simulink model "QArm_with_Dynamic_Model"  (R2024a)
settings: Solver=ode4  StartTime=0.0  StopTime=inf  FixedStep=1/500  RelTol=1e-3  EnableMultiTasking=on
undefined symbols (not defined in the file): HIL, qc_get_step_size
libraries: quarc_library x13
settings Model: SimulationMode=external  ExtModeTrigDuration=10000  Creator=fvranes  LastModifiedBy=mbohra
settings SolverCC: AlgebraicLoopSolver=TrustRegion  PositivePriorityOrder=on
settings DataIOCC: SaveOutput=off  SignalLogging=off  DSMLogging=off  SaveTime=off  ReturnWorkspaceOutputs=off
settings OptimizationCC: ReuseModelBlockBuffer=off
settings DebuggingCC: UnconnectedInputMsg=warning  UnconnectedOutputMsg=warning  UnconnectedLineMsg=warning  ArithmeticOperatorsInVariantConditions=warning
settings ModelReferenceCC: EnableRefExpFcnMdlSchedulingChecks=on
settings SFSimCC: SimUseLocalCustomCode=off  CustomCodeUndefinedFunction=UseInterfaceOnly
settings RTWCC: Description=QUARC Win64 Target Using Toolchain  SystemTargetFile=quarc_win64.tlc  TemplateMakefile=quarc_default_tmf  RTWUseLocalCustomCode=off  Toolchain=QUARC win64 | nmake (64-bit Windows)  BuildConfiguration=Faster Runs  GPUComputeCapability=3.5
settings CodeAppCC: StateflowObjectComments=on
settings STFCustomTargetCC: ConcurrentExecutionCompliant=on  SystemTargetFile=quarc_win64.tlc
settings GRTTargetCC: ParMdlRefBuildCompliant=off  CompOptLevelCompliant=off  CombineOutputUpdateFcns=off  MatFileLogging=off  CPPClassGenCompliant=off  GRTInterface=on  ExtMode=on  ExtModeMexFile=quarc_comm
settings ConfigComp: CovMetricSettings=dswe

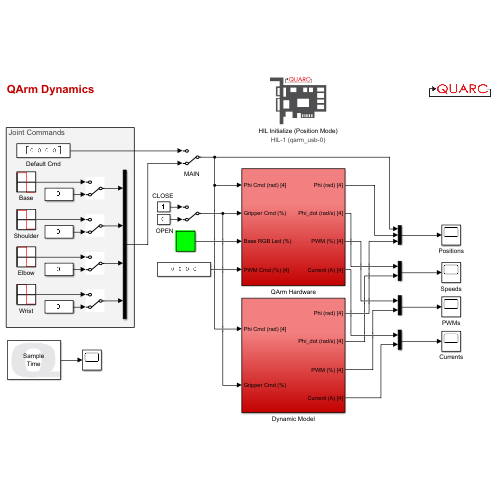
[thumbnail: Simulink's stored preview of the top-level diagram]
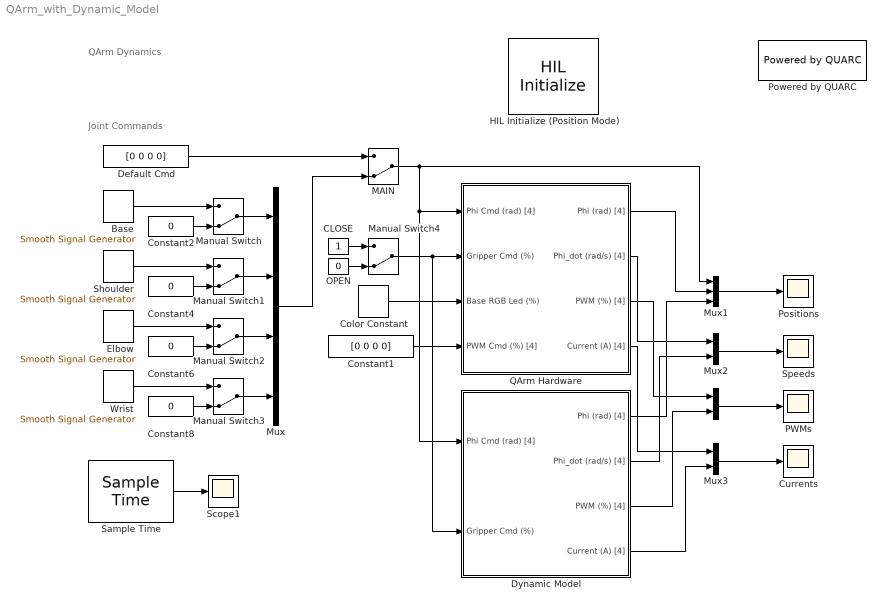
== system QArm_with_Dynamic_Model ==
  note: Joint Commands
  note: QArm Dynamics
  " " : Mux  Inputs=2
  " OPEN" : Constant  Value=0
  Base : quarc_library/Sources/Signals/Smooth Signal Generator  signal_type=Square  source=Internal (dialog parameters)  amplitude=pi/8  frequency=0.125  initial_phase=0  sample_time=qc_get_step_size  output_cos=off
      settings: SourceProductName=QUARC Targets
  "CLOSE " : Constant
  Color Constant : quarc_library/Sources/Signals/Color Constant  color=[0 1 0]
      settings: SourceProductName=QUARC Targets
  Constant1 : Constant  Value=[0 0 0 0]
  Constant{2,4,6,8} (4 alike) : Constant  Value=0
  Currents : Scope
  Default Cmd : Constant  Value=[0 0 0 0]
  Dynamic Model : Subsystem
  Elbow : quarc_library/Sources/Signals/Smooth Signal Generator  signal_type=Square  source=Internal (dialog parameters)  amplitude=pi/8  frequency=0.125  initial_phase=pi  sample_time=qc_get_step_size  output_cos=off
      settings: SourceProductName=QUARC Targets
  HIL Initialize (Position Mode) : quarc_library/Data Acquisition/Generic/Configuration/HIL Initialize  object_name=HIL-1  board_type=qarm_usb  board_number=0  board_options=j0_mode=0;j1_mode=0;j2_mode=0;j3_mode=0;gripper_mode=0;j0_profile_config=0;j0_profile_velocity=1.5708;j0_profile_acceleration=1.0472;j1_profile_config=0;j1_profile_velocity=1.5708;j1_profile_acceleration=1.0472;j2_profile_config=0;j2_profile_velocity=1.5708;j2_profile_acceleration=1.0472;j3_profile_config=0;j3_profile_velocity=1.5708;j3_profile_acceleration=1.0472;  exclusive=off  active=on  hardware_clocks=[0]  clock_modes=[]  initial_clock_frequencies=[]  set_clock_params_at_start=off  set_clock_params_at_switch_in=off  set_clock_frequencies_at_start=off  set_clock_frequencies_at_switch_in=off  analog_input_channels=[5:9]  analog_input_configurations=[]  analog_input_maximums=[]  analog_input_minimums=[]  set_analog_input_params_at_start=off  set_analog_input_params_at_switch_in=off  analog_output_channels=[]  analog_output_maximums=inf  analog_output_minimums=-inf  initial_analog_outputs=[0]  final_analog_outputs=[0]  watchdog_analog_outputs=[]  set_analog_output_params_at_start=off  set_analog_output_params_at_switch_in=off  set_analog_outputs_at_start=off  set_analog_outputs_at_switch_in=off  set_analog_outputs_at_terminate=off  set_analog_outputs_at_switch_out=off  set_analog_outputs_on_watchdog=off  digital_input_channels=[]  digital_output_channels=[]  digital_output_configuration=[]  initial_digital_outputs=[0]  final_digital_outputs=[0]  watchdog_digital_outputs=[0]  set_digital_output_params_at_start=off  set_digital_output_params_at_switch_in=off  set_digital_outputs_at_start=off  set_digital_outputs_at_switch_in=off  set_digital_outputs_at_terminate=off  set_digital_outputs_at_switch_out=off  set_digital_outputs_on_watchdog=off  encoder_channels=[]  quadrature=[]  encoder_filter_frequency=[]  initial_encoder_counts=[]  set_encoder_params_at_start=off  set_encoder_params_at_switch_in=off  set_encoder_counts_at_start=off  set_encoder_counts_at_switch_in=off  pwm_channels=[]  pwm_modes=[]  pwm_frequency=[]  pwm_configuration=[]  pwm_alignment=[]  pwm_polarity=[]  pwm_leading_deadband=[]  pwm_trailing_deadband=[]  initial_pwm_outputs=[]  final_pwm_outputs=[]  watchdog_pwm_outputs=[]  set_pwm_params_at_start=off  set_pwm_params_at_switch_in=off  set_pwm_outputs_at_start=off  set_pwm_outputs_at_switch_in=off  set_pwm_outputs_at_terminate=off  set_pwm_outputs_at_switch_out=off  set_pwm_outputs_on_watchdog=off  other_output_channels=[11005:11008 1000:1004 11000:11003]  initial_other_outputs=[zeros(1,9), ones(1,3)]  final_other_outputs=[1 0 0 0]  watchdog_other_outputs=zeros(1,12)  set_other_outputs_at_start=off  set_other_outputs_at_switch_in=off  set_other_outputs_at_terminate=on  set_other_outputs_at_switch_out=off  set_other_outputs_on_watchdog=off
  MAIN : ManualSwitch  CurrentSetting=0
  Manual Switch{,1..4} (5 alike) : ManualSwitch  CurrentSetting=0
  Mux : Mux
  Mux1 : Mux  Inputs=3
  Mux2 : Mux  Inputs=2
  Mux3 : Mux  Inputs=2
  PWMs : Scope
  Positions : Scope
  Powered by QUARC : quarc_library/Logos/Powered by QUARC
  QArm Hardware : Subsystem
  Sample Time : quarc_library/Sources/Time/Sample Time  Priority=-99  sample_time=qc_get_step_size
  Scope1 : Scope
  Shoulder : quarc_library/Sources/Signals/Smooth Signal Generator  signal_type=Square  source=Internal (dialog parameters)  amplitude=pi/8  frequency=0.125  initial_phase=0  sample_time=qc_get_step_size  output_cos=off
      settings: SourceProductName=QUARC Targets
  Speeds : Scope
  Wrist : quarc_library/Sources/Signals/Smooth Signal Generator  signal_type=Square  source=Internal (dialog parameters)  amplitude=pi/8  frequency=0.125  initial_phase=0  sample_time=qc_get_step_size  output_cos=off
      settings: SourceProductName=QUARC Targets
  wires:
  Color Constant/1 -> QArm Hardware/3(Base RGB Led (%))
  Manual Switch4/1 -> Dynamic Model/2(Gripper Cmd (%)), QArm Hardware/2(Gripper Cmd (%))
  Constant2/1 -> Manual Switch/2
  Constant4/1 -> Manual Switch1/2
  Constant6/1 -> Manual Switch2/2
  Constant8/1 -> Manual Switch3/2
  Wrist/1 -> Manual Switch3/1
  Manual Switch2/1 -> Mux/3
  Manual Switch3/1 -> Mux/4
  Manual Switch1/1 -> Mux/2
  Manual Switch/1 -> Mux/1
  Mux/1 -> MAIN/2
  Default Cmd/1 -> MAIN/1
  MAIN/1 -> Dynamic Model/1(Phi Cmd (rad) [4]), QArm Hardware/1(Phi Cmd (rad) [4]), Mux1/1
  "CLOSE "/1 -> Manual Switch4/1
  QArm Hardware/1(Phi (rad) [4]) -> Mux1/2
  Base/1 -> Manual Switch/1
  Shoulder/1 -> Manual Switch1/1
  Elbow/1 -> Manual Switch2/1
  Constant1/1 -> QArm Hardware/4(PWM Cmd (%) [4])
  Sample Time/1 -> Scope1/1
  " OPEN"/1 -> Manual Switch4/2
  Dynamic Model/1(Phi (rad) [4]) -> Mux1/3
  Mux1/1 -> Positions/1
  Mux2/1 -> Speeds/1
  QArm Hardware/2(Phi_dot (rad/s) [4]) -> Mux2/1
  Dynamic Model/2(Phi_dot (rad/s) [4]) -> Mux2/2
  Mux3/1 -> Currents/1
  QArm Hardware/4(Current (A) [4]) -> Mux3/1
  Dynamic Model/4(Current (A) [4]) -> Mux3/2
  " "/1 -> PWMs/1
  Dynamic Model/3(PWM (%) [4]) -> " "/2
  QArm Hardware/3(PWM (%) [4]) -> " "/1

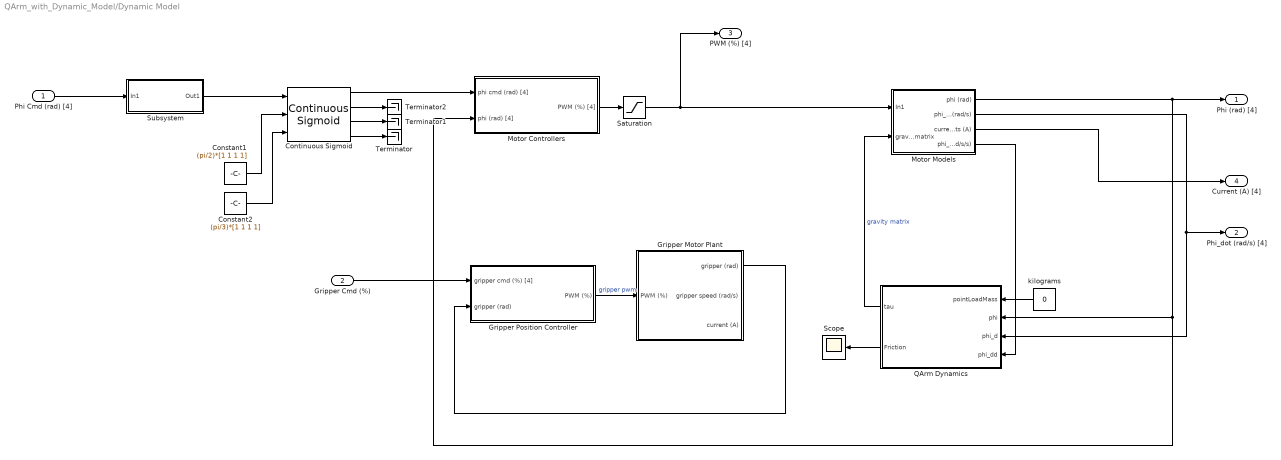
== system QArm_with_Dynamic_Model/Dynamic Model ==
  Phi Cmd (rad) [4] : Inport
  Gripper Cmd (%) : Inport  Port=2
  Constant1 : Constant  Value=(pi/2)*[1 1 1 1]
  Constant2 : Constant  Value=(pi/3)*[1 1 1 1]
  Continuous Sigmoid : quarc_library/Sources/Sigmoids/Continuous Sigmoid  params_source=External (input ports)  max_velocity=10  max_acceleration=10  initial_position=0  initial_velocity=0  hold_off=0.5  input_sample_time=-1  output_sample_time=qc_get_step_size
      settings: SourceProductName=QUARC Targets
  Gripper Motor Plant : Subsystem
  Gripper Position Controller : Subsystem
  Motor Controllers : Subsystem
  Motor Models : Subsystem
  QArm Dynamics : MATLAB Function  TreatAsAtomicUnit=on
  Saturation : Saturate  UpperLimit=[1 1 1 1]  LowerLimit=-1*[1 1 1 1]
  Scope : Scope
  Subsystem : Subsystem
  Terminator : Terminator
  Terminator1 : Terminator
  Terminator2 : Terminator
  kilograms : Constant  Value=0
  Phi (rad) [4] : Outport  VectorParamsAs1DForOutWhenUnconnected=off
  Phi_dot (rad/s) [4] : Outport  Port=2  VectorParamsAs1DForOutWhenUnconnected=off
  PWM (%) [4] : Outport  Port=3  VectorParamsAs1DForOutWhenUnconnected=off
  Current (A) [4] : Outport  Port=4  VectorParamsAs1DForOutWhenUnconnected=off
  wires:
  Gripper Cmd (%)/1 -> Gripper Position Controller/1(gripper cmd (%) [4])
  Gripper Position Controller/1(PWM (%)) -> Gripper Motor Plant/1(PWM (%))  "gripper pwm"
  Gripper Motor Plant/1(gripper (rad)) -> Gripper Position Controller/2(gripper (rad))
  Saturation/1 -> Motor Models/1(In1), PWM (%) [4]/1
  Motor Controllers/1(PWM (%) [4]) -> Saturation/1
  kilograms/1 -> QArm Dynamics/1(pointLoadMass)
  QArm Dynamics/2(Friction) -> Scope/1
  Constant1/1 -> Continuous Sigmoid/2
  Constant2/1 -> Continuous Sigmoid/3
  Continuous Sigmoid/1 -> Motor Controllers/1(phi cmd (rad) [4])
  Continuous Sigmoid/4 -> Terminator/1
  Continuous Sigmoid/3 -> Terminator1/1
  Continuous Sigmoid/2 -> Terminator2/1
  Motor Models/2(phi_dot (rad/s)) -> Phi_dot (rad/s) [4]/1, QArm Dynamics/3(phi_d)
  Motor Models/1(phi (rad)) -> Phi (rad) [4]/1, QArm Dynamics/2(phi), Motor Controllers/2(phi (rad) [4])
  QArm Dynamics/1(tau) -> Motor Models/2(gravity matrix)  "gravity matrix"
  Motor Models/3(currents (A)) -> Current (A) [4]/1
  Motor Models/4(phi_dot_dot (rad/s/s)) -> QArm Dynamics/4(phi_dd)
  Phi Cmd (rad) [4]/1 -> Subsystem/1(In1)
  Subsystem/1(Out1) -> Continuous Sigmoid/1

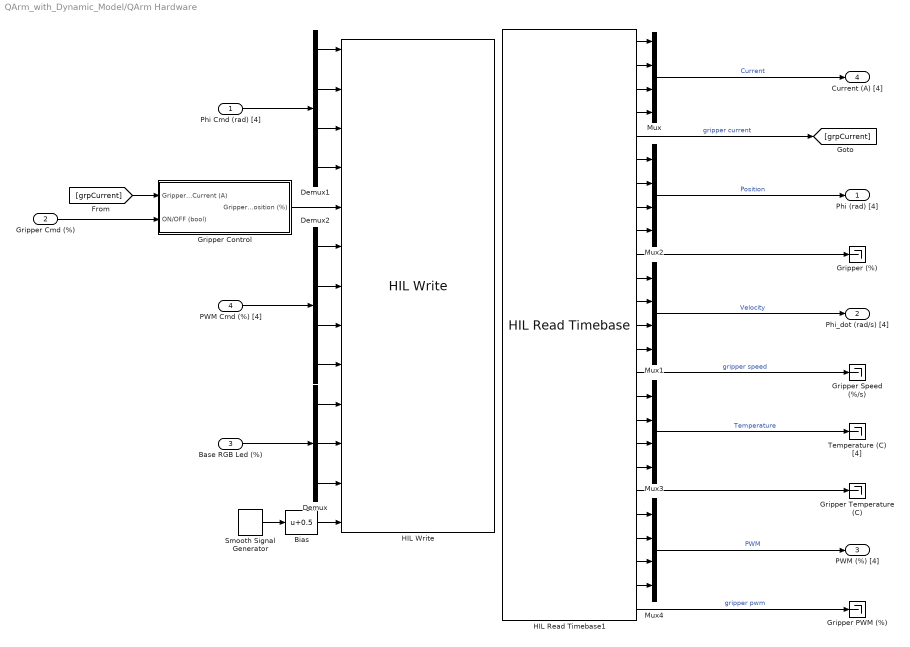
== system QArm_with_Dynamic_Model/QArm Hardware ==
  Phi Cmd (rad) [4] : Inport
  Gripper Cmd (%) : Inport  Port=2
  Base RGB Led (%) : Inport  Port=3
  PWM Cmd (%) [4] : Inport  Port=4
  Bias : Bias  Bias=0.5  SaturateOnIntegerOverflow=off
  Demux : Demux  Outputs=3
  Demux1 : Demux
  Demux2 : Demux
  Gripper (%) : Terminator
  Gripper Control : Subsystem
  Gripper PWM (%) : Terminator
  Gripper Speed (%/s) : Terminator
  Gripper Temperature (C) : Terminator
  HIL Read Timebase1 : quarc_library/Data Acquisition/Generic/Timebases/HIL Read Timebase  object_name=HIL-1  clock=0  analog_channels=[5:9]  encoder_channels=[]  digital_channels=[]  other_channels=[1000:1004 3000:3004 10000:10004 11000:11004]  active=on  vector_output=off  data_type_mode=Inherit via back propagation  encoder_data_type=double  digital_data_type=boolean  overflow_mode=Error on overflow  samples_in_buffer=max(ceil(1/qc_get_step_size), 1)
  HIL Write : quarc_library/Data Acquisition/Generic/Immediate I//O/HIL Write  object_name=HIL-1  analog_channels=[]  pwm_channels=[]  digital_channels=[]  other_channels=[1000:1004 11000:11003 11005:11008]  sample_time=-1  active=on  vector_input=off
  Mux{,1..4} (5 alike) : Mux
  Smooth Signal Generator : quarc_library/Sources/Signals/Smooth Signal Generator  signal_type=Sine  source=Internal (dialog parameters)  amplitude=0.5  frequency=0.5  initial_phase=0  sample_time=qc_get_step_size  output_cos=off
      settings: SourceProductName=QUARC Targets
  Temperature (C) [4] : Terminator
  Phi (rad) [4] : Outport  VectorParamsAs1DForOutWhenUnconnected=off
  Phi_dot (rad/s) [4] : Outport  Port=2  VectorParamsAs1DForOutWhenUnconnected=off
  PWM (%) [4] : Outport  Port=3  VectorParamsAs1DForOutWhenUnconnected=off
  Current (A) [4] : Outport  Port=4  VectorParamsAs1DForOutWhenUnconnected=off
  wires:
  Gripper Cmd (%)/1 -> Gripper Control/2(ON/OFF (bool))
  HIL Read Timebase1/10 -> Gripper (%)/1
  Mux4/1 -> PWM (%) [4]/1  "PWM"
  HIL Read Timebase1/25 -> Gripper PWM (%)/1  "gripper pwm"
  HIL Read Timebase1/24 -> Mux4/4
  HIL Read Timebase1/23 -> Mux4/3
  HIL Read Timebase1/22 -> Mux4/2
  HIL Read Timebase1/21 -> Mux4/1
  Mux2/1 -> Phi (rad) [4]/1  "Position"
  Demux2/4 -> HIL Write/9
  Demux2/3 -> HIL Write/8
  Demux2/2 -> HIL Write/7
  Demux2/1 -> HIL Write/6
  PWM Cmd (%) [4]/1 -> Demux2/1
  Phi Cmd (rad) [4]/1 -> Demux1/1
  Demux1/4 -> HIL Write/4
  Demux1/3 -> HIL Write/3
  Demux1/2 -> HIL Write/2
  Demux1/1 -> HIL Write/1
  Base RGB Led (%)/1 -> Demux/1
  Mux3/1 -> Temperature (C) [4]/1  "Temperature"
  Mux1/1 -> Phi_dot (rad/s) [4]/1  "Velocity"
  Mux/1 -> Current (A) [4]/1  "Current"
  HIL Read Timebase1/20 -> Gripper Temperature (C)/1
  HIL Read Timebase1/1 -> Mux/1
  HIL Read Timebase1/2 -> Mux/2
  HIL Read Timebase1/13 -> Mux1/3
  Demux/2 -> HIL Write/11
  HIL Read Timebase1/19 -> Mux3/4
  Demux/1 -> HIL Write/10
  HIL Read Timebase1/11 -> Mux1/1
  HIL Read Timebase1/16 -> Mux3/1
  HIL Read Timebase1/17 -> Mux3/2
  HIL Read Timebase1/3 -> Mux/3
  Demux/3 -> HIL Write/12
  HIL Read Timebase1/15 -> Gripper Speed (%/s)/1  "gripper speed"
  HIL Read Timebase1/5 -> [grpCurrent]  "gripper current"
  HIL Read Timebase1/7 -> Mux2/2
  HIL Read Timebase1/4 -> Mux/4
  HIL Read Timebase1/12 -> Mux1/2
  HIL Read Timebase1/8 -> Mux2/3
  HIL Read Timebase1/18 -> Mux3/3
  HIL Read Timebase1/6 -> Mux2/1
  HIL Read Timebase1/9 -> Mux2/4
  HIL Read Timebase1/14 -> Mux1/4
  Smooth Signal Generator/1 -> Bias/1
  Bias/1 -> HIL Write/13
  Gripper Control/1(Gripper Position (%)) -> HIL Write/5
  [grpCurrent] -> Gripper Control/1(Gripper Current (A))

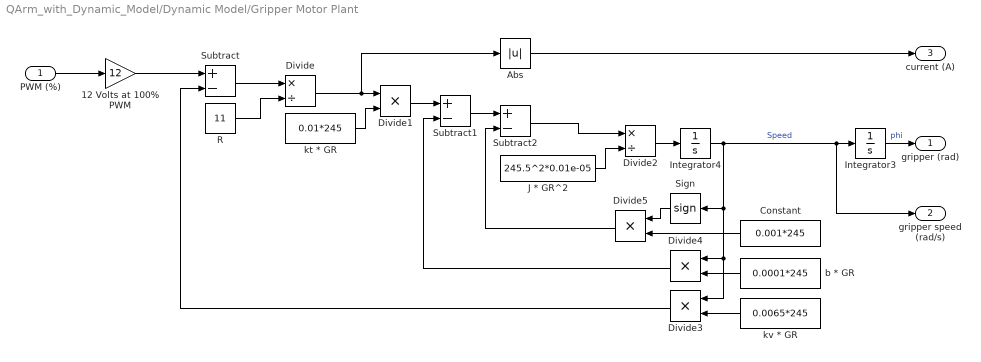
== system QArm_with_Dynamic_Model/Dynamic Model/Gripper Motor Plant ==
  PWM (%) : Inport
  12 Volts at 100% PWM : Gain  Gain=12
  Abs : Abs  SaturateOnIntegerOverflow=off
  Constant : Constant  Value=0.001*245
  Divide : Product  Inputs=*/
  Divide{1,3..5} (4 alike) : Product  Inputs=**
  Divide2 : Product  Inputs=*/
  Integrator3 : Integrator  LimitOutput=on  UpperSaturationLimit=2  LowerSaturationLimit=0
  Integrator4 : Integrator  LimitOutput=on  UpperSaturationLimit=Inf  LowerSaturationLimit=-Inf
  J * GR^2 : Constant  Value=245.5^2*0.01e-05
  R : Constant  Value=11
  Sign : Signum
  Subtract : Sum  Inputs=+-
  Subtract1 : Sum  Inputs=+-
  Subtract2 : Sum  Inputs=+-
  b * GR : Constant  Value=0.0001*245
  kt * GR : Constant  Value=0.01*245
  kv * GR : Constant  Value=0.0065*245
  gripper (rad) : Outport  VectorParamsAs1DForOutWhenUnconnected=off
  gripper speed (rad/s) : Outport  Port=2  VectorParamsAs1DForOutWhenUnconnected=off
  current (A) : Outport  Port=3  VectorParamsAs1DForOutWhenUnconnected=off
  wires:
  Divide4/1 -> Subtract1/2
  Divide2/1 -> Integrator4/1
  Integrator3/1 -> gripper (rad)/1  "phi"
  b * GR/1 -> Divide4/2
  kv * GR/1 -> Divide3/2
  PWM (%)/1 -> 12 Volts at 100% PWM/1
  Subtract1/1 -> Subtract2/1
  J * GR^2/1 -> Divide2/2
  Divide1/1 -> Subtract1/1
  Divide3/1 -> Subtract/2
  Divide/1 -> Divide1/1, Abs/1
  kt * GR/1 -> Divide1/2
  Subtract/1 -> Divide/1
  R/1 -> Divide/2
  Sign/1 -> Divide5/1
  Constant/1 -> Divide5/2
  Integrator4/1 -> Integrator3/1, gripper speed (rad/s)/1, Sign/1, Divide3/1, Divide4/1  "Speed"
  Divide5/1 -> Subtract2/2
  Subtract2/1 -> Divide2/1
  12 Volts at 100% PWM/1 -> Subtract/1
  Abs/1 -> current (A)/1

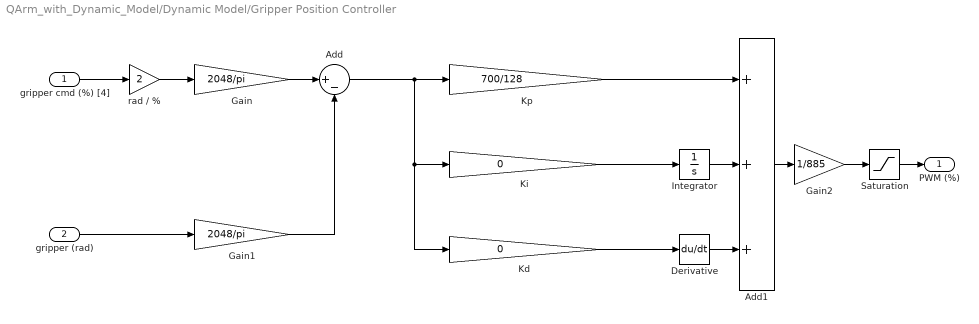
== system QArm_with_Dynamic_Model/Dynamic Model/Gripper Position Controller ==
  gripper cmd (%) [4] : Inport
  gripper (rad) : Inport  Port=2
  Add : Sum  Inputs=|+-
  Add1 : Sum  Inputs=+++
  Derivative : Derivative
  Gain : Gain  Gain=2048/pi
  Gain1 : Gain  Gain=2048/pi
  Gain2 : Gain  Gain=1/885
  Integrator : Integrator
  Kd : Gain  Gain=0
  Ki : Gain  Gain=0
  Kp : Gain  Gain=700/128
  Saturation : Saturate  UpperLimit=1  LowerLimit=-1
  rad / % : Gain  Gain=2
  PWM (%) : Outport  VectorParamsAs1DForOutWhenUnconnected=off
  wires:
  Kd/1 -> Derivative/1
  Ki/1 -> Integrator/1
  Saturation/1 -> PWM (%)/1
  Derivative/1 -> Add1/3
  Integrator/1 -> Add1/2
  Add/1 -> Kp/1, Ki/1, Kd/1
  Add1/1 -> Gain2/1
  gripper cmd (%) [4]/1 -> rad / %/1
  Kp/1 -> Add1/1
  rad / %/1 -> Gain/1
  gripper (rad)/1 -> Gain1/1
  Gain/1 -> Add/1
  Gain1/1 -> Add/2
  Gain2/1 -> Saturation/1

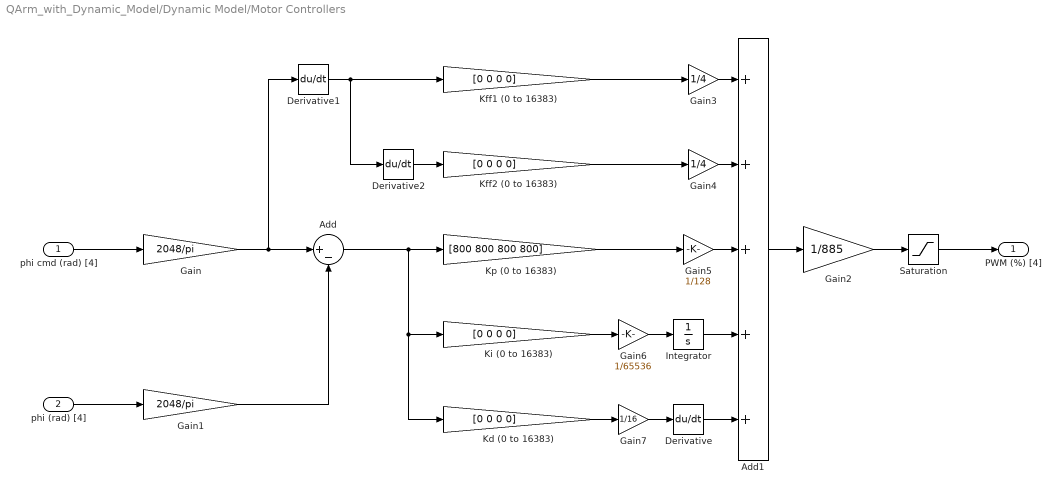
== system QArm_with_Dynamic_Model/Dynamic Model/Motor Controllers ==
  phi cmd (rad) [4] : Inport
  phi (rad) [4] : Inport  Port=2
  Add : Sum  Inputs=|+-
  Add1 : Sum  Inputs=+++++
  Derivative : Derivative
  Derivative1 : Derivative
  Derivative2 : Derivative
  Gain : Gain  Gain=2048/pi
  Gain1 : Gain  Gain=2048/pi
  Gain2 : Gain  Gain=1/885
  Gain3 : Gain  Gain=1/4
  Gain4 : Gain  Gain=1/4
  Gain5 : Gain  Gain=1/128
  Gain6 : Gain  Gain=1/65536
  Gain7 : Gain  Gain=1/16
  Integrator : Integrator
  Kd (0 to 16383) : Gain  Gain=[0 0 0 0]
  Kff1 (0 to 16383) : Gain  Gain=[0 0 0 0]
  Kff2 (0 to 16383) : Gain  Gain=[0 0 0 0]
  Ki (0 to 16383) : Gain  Gain=[0 0 0 0]
  Kp (0 to 16383) : Gain  Gain=[800 800 800 800]
  Saturation : Saturate  UpperLimit=[1 1 1 1]  LowerLimit=-1*[1 1 1 1]
  PWM (%) [4] : Outport  VectorParamsAs1DForOutWhenUnconnected=off
  wires:
  phi cmd (rad) [4]/1 -> Gain/1
  phi (rad) [4]/1 -> Gain1/1
  Gain2/1 -> Saturation/1
  Gain1/1 -> Add/2
  Ki (0 to 16383)/1 -> Gain6/1
  Kd (0 to 16383)/1 -> Gain7/1
  Add/1 -> Kd (0 to 16383)/1, Ki (0 to 16383)/1, Kp (0 to 16383)/1
  Integrator/1 -> Add1/4
  Derivative/1 -> Add1/5
  Add1/1 -> Gain2/1
  Gain/1 -> Derivative1/1, Add/1
  Kff2 (0 to 16383)/1 -> Gain4/1
  Derivative1/1 -> Derivative2/1, Kff1 (0 to 16383)/1
  Derivative2/1 -> Kff2 (0 to 16383)/1
  Kff1 (0 to 16383)/1 -> Gain3/1
  Kp (0 to 16383)/1 -> Gain5/1
  Saturation/1 -> PWM (%) [4]/1
  Gain3/1 -> Add1/1
  Gain4/1 -> Add1/2
  Gain5/1 -> Add1/3
  Gain6/1 -> Integrator/1
  Gain7/1 -> Derivative/1

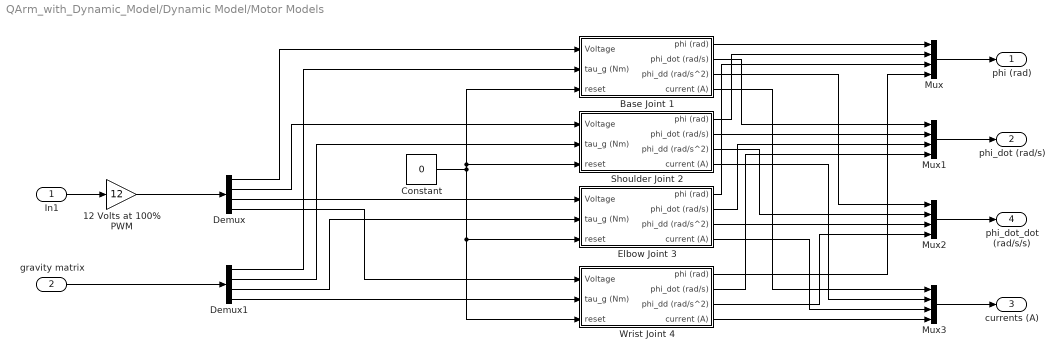
== system QArm_with_Dynamic_Model/Dynamic Model/Motor Models ==
  In1 : Inport
  gravity matrix : Inport  Port=2
  12 Volts at 100% PWM : Gain  Gain=12
  Base Joint 1 : Subsystem
  Constant : Constant  Value=0
  Demux : Demux
  Demux1 : Demux
  Elbow Joint 3 : Subsystem
  Mux{,1..3} (4 alike) : Mux
  Shoulder Joint 2 : Subsystem
  Wrist Joint 4 : Subsystem
  phi (rad) : Outport
  phi_dot (rad/s) : Outport  Port=2
  currents (A) : Outport  Port=3
  phi_dot_dot (rad/s/s) : Outport  Port=4
  wires:
  Demux/1 -> Base Joint 1/1(Voltage)
  Elbow Joint 3/1(phi (rad)) -> Mux/3
  Wrist Joint 4/4(current (A)) -> Mux3/4
  Demux/4 -> Wrist Joint 4/1(Voltage)
  Shoulder Joint 2/4(current (A)) -> Mux3/2
  Constant/1 -> Wrist Joint 4/3(reset), Elbow Joint 3/3(reset), Base Joint 1/3(reset), Shoulder Joint 2/3(reset)
  Shoulder Joint 2/3(phi_dd (rad/s^2)) -> Mux2/2
  Demux1/4 -> Wrist Joint 4/2(tau_g (Nm))
  Elbow Joint 3/4(current (A)) -> Mux3/3
  Shoulder Joint 2/1(phi (rad)) -> Mux/2
  12 Volts at 100% PWM/1 -> Demux/1
  Wrist Joint 4/2(phi_dot (rad/s)) -> Mux1/4
  Wrist Joint 4/1(phi (rad)) -> Mux/4
  Elbow Joint 3/2(phi_dot (rad/s)) -> Mux1/3
  Wrist Joint 4/3(phi_dd (rad/s^2)) -> Mux2/4
  gravity matrix/1 -> Demux1/1
  Base Joint 1/2(phi_dot (rad/s)) -> Mux1/1
  Elbow Joint 3/3(phi_dd (rad/s^2)) -> Mux2/3
  Base Joint 1/4(current (A)) -> Mux3/1
  Base Joint 1/1(phi (rad)) -> Mux/1
  Demux/3 -> Elbow Joint 3/1(Voltage)
  Demux1/3 -> Elbow Joint 3/2(tau_g (Nm))
  Base Joint 1/3(phi_dd (rad/s^2)) -> Mux2/1
  Demux1/2 -> Shoulder Joint 2/2(tau_g (Nm))
  Demux/2 -> Shoulder Joint 2/1(Voltage)
  Shoulder Joint 2/2(phi_dot (rad/s)) -> Mux1/2
  Mux1/1 -> phi_dot (rad/s)/1
  Demux1/1 -> Base Joint 1/2(tau_g (Nm))
  Mux3/1 -> currents (A)/1
  In1/1 -> 12 Volts at 100% PWM/1
  Mux/1 -> phi (rad)/1
  Mux2/1 -> phi_dot_dot (rad/s/s)/1

== system QArm_with_Dynamic_Model/Dynamic Model/Subsystem ==
  In1 : Inport
  Demux : Demux
  Mux : Mux
  Transfer Fcn{,1..3} (4 alike) : TransferFcn  Denominator=[0.4 1]
  Out1 : Outport
  wires:
  In1/1 -> Demux/1
  Mux/1 -> Out1/1
  Demux/1 -> Transfer Fcn/1
  Demux/2 -> Transfer Fcn1/1
  Demux/3 -> Transfer Fcn2/1
  Demux/4 -> Transfer Fcn3/1
  Transfer Fcn1/1 -> Mux/2
  Transfer Fcn2/1 -> Mux/3
  Transfer Fcn/1 -> Mux/1
  Transfer Fcn3/1 -> Mux/4

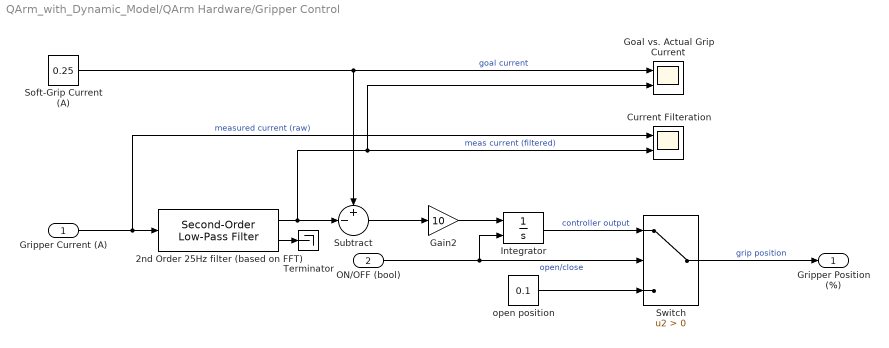
== system QArm_with_Dynamic_Model/QArm Hardware/Gripper Control ==
  Gripper Current (A) : Inport
  ON/OFF (bool) : Inport  Port=2
  2nd Order 25Hz filter (based on FFT) : quarc_library/Continuous/Second-Order Low-Pass Filter  params_source=Internal (dialog parameters)  input_width=25*2*pi  input_zeta=1  input_init=0
  Current Filteration : Scope  NumInputPorts=2
  Gain2 : Gain  Gain=10
  Goal vs. Actual Grip Current : Scope  NumInputPorts=2
  Integrator : Integrator  ExternalReset=either  InitialCondition=0.1  LimitOutput=on  UpperSaturationLimit=0.9  LowerSaturationLimit=0.1
  Soft-Grip Current (A) : Constant  Value=0.25
  Subtract : Sum  Inputs=+-|
  Switch : Switch  Criteria=u2 > Threshold  SaturateOnIntegerOverflow=off  InputSameDT=off
  Terminator : Terminator
  open position : Constant  Value=0.1
  Gripper Position (%) : Outport  VectorParamsAs1DForOutWhenUnconnected=off
  wires:
  Gripper Current (A)/1 -> 2nd Order 25Hz filter (based on FFT)/1, Current Filteration/1  "measured current (raw)"
  ON/OFF (bool)/1 -> Switch/2, Integrator/2  "open/close"
  open position/1 -> Switch/3
  Switch/1 -> Gripper Position (%)/1  "grip position"
  Soft-Grip Current (A)/1 -> Subtract/1, Goal vs. Actual Grip Current/1  "goal current"
  2nd Order 25Hz filter (based on FFT)/1 -> Subtract/2, Current Filteration/2, Goal vs. Actual Grip Current/2  "meas current (filtered)"
  Subtract/1 -> Gain2/1
  Integrator/1 -> Switch/1  "controller output"
  Gain2/1 -> Integrator/1
  2nd Order 25Hz filter (based on FFT)/2 -> Terminator/1

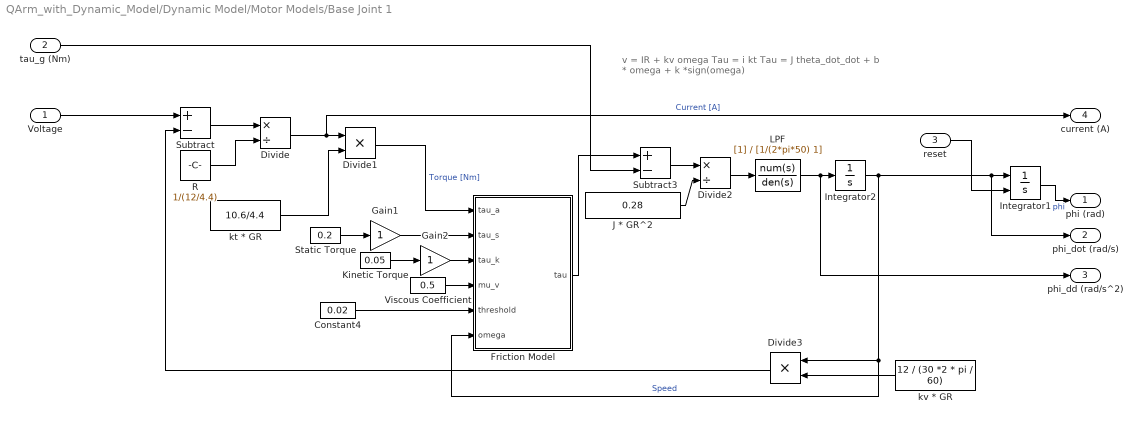
== system QArm_with_Dynamic_Model/Dynamic Model/Motor Models/Base Joint 1 ==
  note: v = IR + kv omega
      | Tau = i kt
      | Tau = J theta_dot_dot + b * omega + k *sign(omega)
  Voltage : Inport
  tau_g (Nm) : Inport  Port=2
  reset : Inport  Port=3
  Constant4 : Constant  Value=0.02
  Divide : Product  Inputs=*/
  Divide1 : Product  Inputs=**
  Divide2 : Product  Inputs=*/
  Divide3 : Product  Inputs=**
  Friction Model : MATLAB Function  TreatAsAtomicUnit=on
  Gain1 : Gain
  Gain2 : Gain
  Integrator1 : Integrator  ExternalReset=rising  LimitOutput=on  UpperSaturationLimit=pi*[170]/180  LowerSaturationLimit=pi*[-170]/180
  Integrator2 : Integrator  LimitOutput=on  UpperSaturationLimit=pi/2  LowerSaturationLimit=-pi/2
  J * GR^2 : Constant  Value=0.28
  Kinetic Torque : Constant  Value=0.05
  LPF : TransferFcn  Denominator=[1/(2*pi*50) 1]
  R : Constant  Value=1/(12/4.4)
  Static Torque : Constant  Value=0.2
  Subtract : Sum  Inputs=+-
  Subtract3 : Sum  Inputs=+-
  Viscous Coefficient : Constant  Value=0.5
  kt * GR : Constant  Value=10.6/4.4
  kv * GR : Constant  Value=12 / (30 *2 * pi / 60)
  phi (rad) : Outport  VectorParamsAs1DForOutWhenUnconnected=off
  phi_dot (rad/s) : Outport  Port=2  VectorParamsAs1DForOutWhenUnconnected=off
  phi_dd (rad/s^2) : Outport  Port=3  VectorParamsAs1DForOutWhenUnconnected=off
  current (A) : Outport  Port=4  VectorParamsAs1DForOutWhenUnconnected=off
  wires:
  R/1 -> Divide/2
  Subtract/1 -> Divide/1
  kt * GR/1 -> Divide1/2
  Divide/1 -> current (A)/1, Divide1/1  "Current [A]"
  Divide3/1 -> Subtract/2
  Divide1/1 -> Friction Model/1(tau_a)  "Torque [Nm]"
  J * GR^2/1 -> Divide2/2
  Voltage/1 -> Subtract/1
  kv * GR/1 -> Divide3/2
  Integrator1/1 -> phi (rad)/1  "phi"
  Divide2/1 -> LPF/1
  Integrator2/1 -> Friction Model/6(omega), Divide3/1, phi_dot (rad/s)/1, Integrator1/1  "Speed"
  Friction Model/1(tau) -> Subtract3/1
  Subtract3/1 -> Divide2/1
  tau_g (Nm)/1 -> Subtract3/2
  reset/1 -> Integrator1/2
  Viscous Coefficient/1 -> Friction Model/4(mu_v)
  Kinetic Torque/1 -> Gain2/1
  Gain2/1 -> Friction Model/3(tau_k)
  Gain1/1 -> Friction Model/2(tau_s)
  Constant4/1 -> Friction Model/5(threshold)
  Static Torque/1 -> Gain1/1
  LPF/1 -> phi_dd (rad/s^2)/1, Integrator2/1

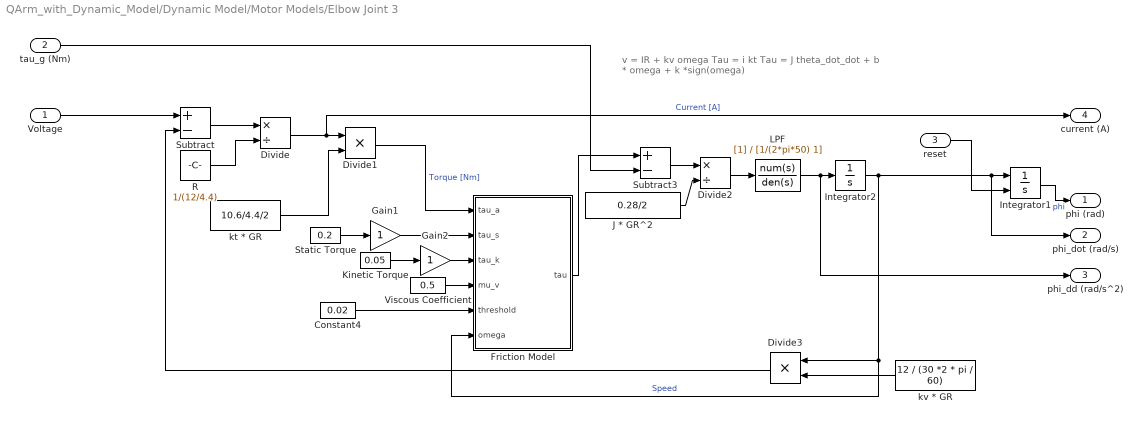
== system QArm_with_Dynamic_Model/Dynamic Model/Motor Models/Elbow Joint 3 ==
  note: v = IR + kv omega
      | Tau = i kt
      | Tau = J theta_dot_dot + b * omega + k *sign(omega)
  Voltage : Inport
  tau_g (Nm) : Inport  Port=2
  reset : Inport  Port=3
  Constant4 : Constant  Value=0.02
  Divide : Product  Inputs=*/
  Divide1 : Product  Inputs=**
  Divide2 : Product  Inputs=*/
  Divide3 : Product  Inputs=**
  Friction Model : MATLAB Function  TreatAsAtomicUnit=on
  Gain1 : Gain
  Gain2 : Gain
  Integrator1 : Integrator  ExternalReset=rising  InitialCondition=-pi*[0]/180  LimitOutput=on  UpperSaturationLimit=pi*[75]/180  LowerSaturationLimit=pi*[-95]/180
  Integrator2 : Integrator  LimitOutput=on  UpperSaturationLimit=pi/2  LowerSaturationLimit=-pi/2
  J * GR^2 : Constant  Value=0.28/2
  Kinetic Torque : Constant  Value=0.05
  LPF : TransferFcn  Denominator=[1/(2*pi*50) 1]
  R : Constant  Value=1/(12/4.4)
  Static Torque : Constant  Value=0.2
  Subtract : Sum  Inputs=+-
  Subtract3 : Sum  Inputs=+-
  Viscous Coefficient : Constant  Value=0.5
  kt * GR : Constant  Value=10.6/4.4/2
  kv * GR : Constant  Value=12 / (30 *2 * pi / 60)
  phi (rad) : Outport  VectorParamsAs1DForOutWhenUnconnected=off
  phi_dot (rad/s) : Outport  Port=2  VectorParamsAs1DForOutWhenUnconnected=off
  phi_dd (rad/s^2) : Outport  Port=3  VectorParamsAs1DForOutWhenUnconnected=off
  current (A) : Outport  Port=4  VectorParamsAs1DForOutWhenUnconnected=off
  wires:
  R/1 -> Divide/2
  Subtract/1 -> Divide/1
  kt * GR/1 -> Divide1/2
  Divide/1 -> current (A)/1, Divide1/1  "Current [A]"
  Divide3/1 -> Subtract/2
  Divide1/1 -> Friction Model/1(tau_a)  "Torque [Nm]"
  J * GR^2/1 -> Divide2/2
  Voltage/1 -> Subtract/1
  kv * GR/1 -> Divide3/2
  Integrator1/1 -> phi (rad)/1  "phi"
  Divide2/1 -> LPF/1
  Integrator2/1 -> Friction Model/6(omega), Divide3/1, Integrator1/1, phi_dot (rad/s)/1  "Speed"
  Friction Model/1(tau) -> Subtract3/1
  Subtract3/1 -> Divide2/1
  tau_g (Nm)/1 -> Subtract3/2
  reset/1 -> Integrator1/2
  Viscous Coefficient/1 -> Friction Model/4(mu_v)
  Kinetic Torque/1 -> Gain2/1
  Gain2/1 -> Friction Model/3(tau_k)
  Gain1/1 -> Friction Model/2(tau_s)
  Constant4/1 -> Friction Model/5(threshold)
  Static Torque/1 -> Gain1/1
  LPF/1 -> phi_dd (rad/s^2)/1, Integrator2/1

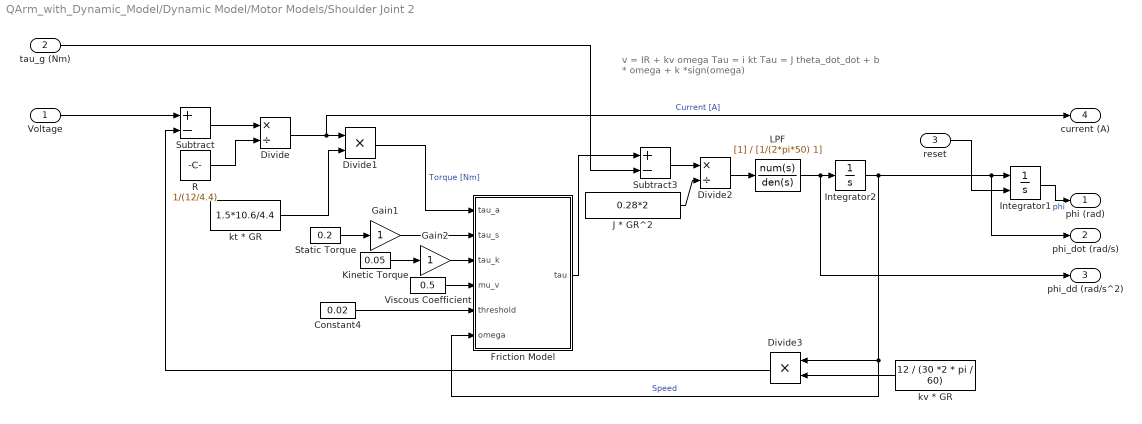
== system QArm_with_Dynamic_Model/Dynamic Model/Motor Models/Shoulder Joint 2 ==
  note: v = IR + kv omega
      | Tau = i kt
      | Tau = J theta_dot_dot + b * omega + k *sign(omega)
  Voltage : Inport
  tau_g (Nm) : Inport  Port=2
  reset : Inport  Port=3
  Constant4 : Constant  Value=0.02
  Divide : Product  Inputs=*/
  Divide1 : Product  Inputs=**
  Divide2 : Product  Inputs=*/
  Divide3 : Product  Inputs=**
  Friction Model : MATLAB Function  TreatAsAtomicUnit=on
  Gain1 : Gain
  Gain2 : Gain
  Integrator1 : Integrator  ExternalReset=rising  LimitOutput=on  UpperSaturationLimit=pi*[85]/180  LowerSaturationLimit=pi*[-85]/180
  Integrator2 : Integrator  LimitOutput=on  UpperSaturationLimit=pi/2  LowerSaturationLimit=-pi/2
  J * GR^2 : Constant  Value=0.28*2
  Kinetic Torque : Constant  Value=0.05
  LPF : TransferFcn  Denominator=[1/(2*pi*50) 1]
  R : Constant  Value=1/(12/4.4)
  Static Torque : Constant  Value=0.2
  Subtract : Sum  Inputs=+-
  Subtract3 : Sum  Inputs=+-
  Viscous Coefficient : Constant  Value=0.5
  kt * GR : Constant  Value=1.5*10.6/4.4
  kv * GR : Constant  Value=12 / (30 *2 * pi / 60)
  phi (rad) : Outport  VectorParamsAs1DForOutWhenUnconnected=off
  phi_dot (rad/s) : Outport  Port=2  VectorParamsAs1DForOutWhenUnconnected=off
  phi_dd (rad/s^2) : Outport  Port=3  VectorParamsAs1DForOutWhenUnconnected=off
  current (A) : Outport  Port=4  VectorParamsAs1DForOutWhenUnconnected=off
  wires:
  LPF/1 -> Integrator2/1, phi_dd (rad/s^2)/1
  Static Torque/1 -> Gain1/1
  Constant4/1 -> Friction Model/5(threshold)
  Gain1/1 -> Friction Model/2(tau_s)
  Gain2/1 -> Friction Model/3(tau_k)
  Kinetic Torque/1 -> Gain2/1
  Viscous Coefficient/1 -> Friction Model/4(mu_v)
  reset/1 -> Integrator1/2
  tau_g (Nm)/1 -> Subtract3/2
  Subtract3/1 -> Divide2/1
  Friction Model/1(tau) -> Subtract3/1
  Integrator2/1 -> Integrator1/1, phi_dot (rad/s)/1, Divide3/1, Friction Model/6(omega)  "Speed"
  Divide2/1 -> LPF/1
  Integrator1/1 -> phi (rad)/1  "phi"
  kv * GR/1 -> Divide3/2
  Voltage/1 -> Subtract/1
  J * GR^2/1 -> Divide2/2
  Divide1/1 -> Friction Model/1(tau_a)  "Torque [Nm]"
  Divide3/1 -> Subtract/2
  Divide/1 -> Divide1/1, current (A)/1  "Current [A]"
  kt * GR/1 -> Divide1/2
  Subtract/1 -> Divide/1
  R/1 -> Divide/2

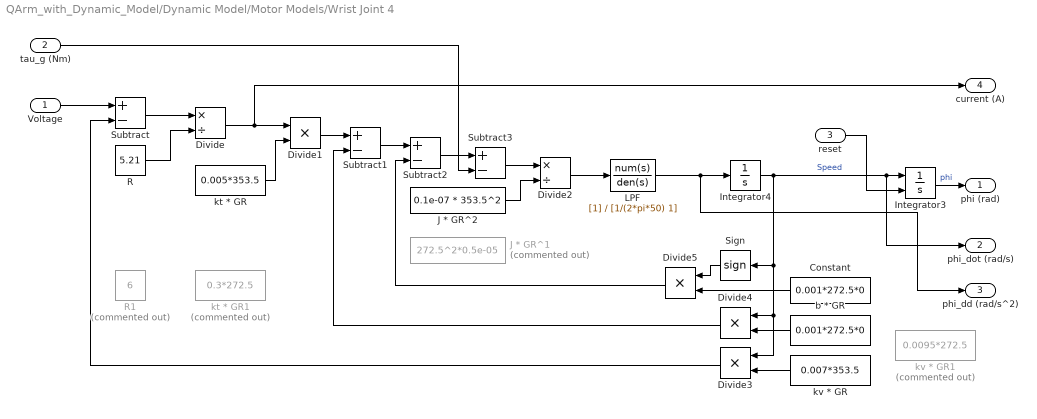
== system QArm_with_Dynamic_Model/Dynamic Model/Motor Models/Wrist Joint 4 ==
  Voltage : Inport
  tau_g (Nm) : Inport  Port=2
  reset : Inport  Port=3
  Constant : Constant  Value=0.001*272.5*0
  Divide : Product  Inputs=*/
  Divide{1,3..5} (4 alike) : Product  Inputs=**
  Divide2 : Product  Inputs=*/
  Integrator3 : Integrator  ExternalReset=rising  LimitOutput=on  UpperSaturationLimit=pi*[167.5]/180  LowerSaturationLimit=pi*[-167.5]/180
  Integrator4 : Integrator  LimitOutput=on  UpperSaturationLimit=pi  LowerSaturationLimit=-pi
  J * GR^1 : Constant  Commented=on  Value=272.5^2*0.5e-05
  J * GR^2 : Constant  Value=0.1e-07 * 353.5^2
  LPF : TransferFcn  Denominator=[1/(2*pi*50) 1]
  R : Constant  Value=5.21
  R1 : Constant  Commented=on  Value=6
  Sign : Signum
  Subtract{,1..3} (4 alike) : Sum  Inputs=+-
  b * GR : Constant  Value=0.001*272.5*0
  kt * GR : Constant  Value=0.005*353.5
  kt * GR1 : Constant  Commented=on  Value=0.3*272.5
  kv * GR : Constant  Value=0.007*353.5
  kv * GR1 : Constant  Commented=on  Value=0.0095*272.5
  phi (rad) : Outport  VectorParamsAs1DForOutWhenUnconnected=off
  phi_dot (rad/s) : Outport  Port=2  VectorParamsAs1DForOutWhenUnconnected=off
  phi_dd (rad/s^2) : Outport  Port=3  VectorParamsAs1DForOutWhenUnconnected=off
  current (A) : Outport  Port=4  VectorParamsAs1DForOutWhenUnconnected=off
  wires:
  Divide4/1 -> Subtract1/2
  LPF/1 -> Integrator4/1, phi_dd (rad/s^2)/1
  Integrator3/1 -> phi (rad)/1  "phi"
  b * GR/1 -> Divide4/2
  kv * GR/1 -> Divide3/2
  Voltage/1 -> Subtract/1
  Subtract1/1 -> Subtract2/1
  J * GR^2/1 -> Divide2/2
  Divide1/1 -> Subtract1/1
  Divide3/1 -> Subtract/2
  Divide/1 -> Divide1/1, current (A)/1
  kt * GR/1 -> Divide1/2
  Subtract/1 -> Divide/1
  R/1 -> Divide/2
  Sign/1 -> Divide5/1
  Constant/1 -> Divide5/2
  Integrator4/1 -> Integrator3/1, phi_dot (rad/s)/1, Sign/1, Divide3/1, Divide4/1  "Speed"
  Divide5/1 -> Subtract2/2
  Subtract3/1 -> Divide2/1
  Subtract2/1 -> Subtract3/1
  tau_g (Nm)/1 -> Subtract3/2
  reset/1 -> Integrator3/2
  Divide2/1 -> LPF/1

== matlab function QArm_with_Dynamic_Model/Dynamic Model/Motor Models/Shoulder Joint 2/Friction Model ==
  data: tau_a input; tau output; tau_s input; tau_k input; mu_v input; threshold input; omega input
function tau = fcn(tau_a, tau_s, tau_k, mu_v, threshold, omega)

% Friction Model:
% tau           - output torque
% tau_a         - applied torque
% tau_s         - static friction torque
% tau_k         - kinetic friction torque
% tau_v         - viscous friction torque
% threshold     - threshold under which you want omega to be considered 0
% omega         - angular speed

% v1.0 Murtaza Bohra
not_moving = 0;
if abs(omega) <= threshold
    not_moving = 1;
end

if (abs(tau_a) < tau_s)&&(not_moving)
    tau = 0;
else
    tau = tau_a - tau_k*sign(omega) - mu_v*omega;
end

== matlab function QArm_with_Dynamic_Model/Dynamic Model/Motor Models/Elbow Joint 3/Friction Model ==
  data: tau_a input; tau output; tau_s input; tau_k input; mu_v input; threshold input; omega input
function tau = fcn(tau_a, tau_s, tau_k, mu_v, threshold, omega)

% Friction Model:
% tau           - output torque
% tau_a         - applied torque
% tau_s         - static friction torque
% tau_k         - kinetic friction torque
% tau_v         - viscous friction torque
% threshold     - threshold under which you want omega to be considered 0
% omega         - angular speed

% v1.0 Murtaza Bohra
not_moving = 0;
if abs(omega) <= threshold
    not_moving = 1;
end

if (abs(tau_a) < tau_s)&&(not_moving)
    tau = 0;
else
    tau = tau_a - tau_k*sign(omega) - mu_v*omega;
end

== matlab function QArm_with_Dynamic_Model/Dynamic Model/Motor Models/Base Joint 1/Friction Model ==
  data: tau_a input; tau output; tau_s input; tau_k input; mu_v input; threshold input; omega input
function tau = fcn(tau_a, tau_s, tau_k, mu_v, threshold, omega)

% Friction Model:
% tau           - output torque
% tau_a         - applied torque
% tau_s         - static friction torque
% tau_k         - kinetic friction torque
% tau_v         - viscous friction torque
% threshold     - threshold under which you want omega to be considered 0
% omega         - angular speed

% v1.0 Murtaza Bohra
not_moving = 0;
if abs(omega) <= threshold
    not_moving = 1;
end

if (abs(tau_a) < tau_s)&&(not_moving)
    tau = 0;
else
    tau = tau_a - tau_k*sign(omega) - mu_v*omega;
end

== matlab function QArm_with_Dynamic_Model/Dynamic Model/QArm Dynamics ==
  data: pointLoadMass input; phi input; phi_d input; phi_dd input; tau output; Friction output
function [tau,Friction]   = f_QArm_Dynamics(pointLoadMass, phi, phi_d, phi_dd)
% Code updated by Leonam Pecly - November 10, 2021
% Based on code provided by Quanser

%%
g = 9.80665;

%% Manipulator parameters:
L1 = 0.1400;
L2 = 0.3500;
L3 = 0.0500;
L4 = 0.2500;
L5 = 0.1500;
beta = atan(L3/L2);

%% Alternate parameters
l1 = L1;                        % lambda 1
l2 = sqrt(L2^2 + L3^2);         % lambda 2
l3 = L4 + L5;                   % lambda 3

theta = phi - [0; pi/2-beta; beta; 0];
theta_d = phi_d;
theta_dd = phi_dd;

%% Dynamic Parameters
m1 = 0.7906;
m2 = 0.4591;
m3 = 0.269;
m4 = 0.257;
mL = pointLoadMass;
I1A = 1.489e-3;
I1L = 1;
I2A = 1.922e-4;
I2L = 9.61e-3;
I3A = 2.679e-4;
I3L = 2.069e-3;
I4A = 5.528e-4;
I4L = 1.12e-3;
% lc1 = l1/3;
% lc2 = l2/2;
% lc3 = L4/2;
% lc4 = L5/2;

lc1 = 0.0399;
lc2 = 0.1071;
lc3 = 0.1561;
lc4 = 0.0998;

%% Dynamic Matrices
% Inertia Matrix
M11 = I1A + m2*(l2 - lc2)^2*cos(theta(2))^2 + I2A*sin(theta(2))^2 + I2L*cos(theta(2))^2 + m3*l2^2*cos(theta(2))^2 + m3*lc3^2*sin(theta(2)+theta(3))^2 - 2*m3*l2*lc3*cos(theta(2))*sin(theta(2)+theta(3))...
    + I3L*sin(theta(2)+theta(3))^2 + I3A*cos(theta(2)+theta(3))^2 + m4*(l3 - lc4)^2*sin(theta(2)+theta(3))^2 + m4*l2^2*cos(theta(2))^2 - 2*m4*(l3-lc4)*l2*cos(theta(2))*sin(theta(2)+theta(3))...
    + I4L*sin(theta(2)+theta(3))^2 + I4A*cos(theta(2)+theta(3))^2 + mL*l3^2*sin(theta(2)+theta(3))^2 + mL*l2^2*cos(theta(2))^2 - 2*mL*l2*l3*cos(theta(2))*sin(theta(2)+theta(3));
M14 = -I4A*cos(theta(2)+theta(3));
M22 = m2*(l2-lc2)^2 + I2L + m3*l2^2+m3*lc3^2 - 2*m3*l2*lc3*sin(theta(3)) + I3L + m4*(l2+l3-lc4)^2 + I4L + mL*l2^2 + mL*l3^2 - 2*mL*l2*l3*sin(theta(3));
M23 = m3*lc3^2 - m3*lc3*l2*sin(theta(3)) + I3L + m4*(l3 - lc4 - l2*sin(theta(3)))*(l3 - lc4) + I4L - mL*(l3^2 - l2*l3*sin(theta(3)));
M32 = m3*lc3^2 - m3*lc3*l2*sin(theta(3)) + I3L + m4*(l3 - lc4 - l2*sin(theta(3)))*(l3 - lc4) + I4L - mL*(l3^2 - l2*l3*sin(theta(3)));
M33 = m3*lc3^2 + I3L + m4*(lc4 - l3)^2 + I4L + mL*l3^2;
M41 = -I4A*cos(theta(2)+theta(3));
M44 = I4A;
M = [M11, 0, 0, M14; 0, M22, M23, 0; 0, M32, M33, 0; M41, 0, 0, M44];

% Coriolis Matrix
B11 = -2*m2*(l2-lc2)^2*sin(theta(2))*cos(theta(2)) + 2*I2A*sin(theta(2))*cos(theta(2)) - 2*I2L*sin(theta(2))*cos(theta(2)) - 2*m3*l2^2*sin(theta(2))*cos(theta(2))...
     + 2*m3*lc3^2*sin(theta(2)+theta(3))*cos(theta(2)+theta(3)) + 2*m3*l2*lc3*sin(theta(2))*sin(theta(2)+theta(3)) - 2*m3*l2*lc3*cos(theta(2))*cos(theta(2)+theta(3))...
     + 2*I3L*sin(theta(2)+theta(3))*cos(theta(2)+theta(3)) - 2*I3A*sin(theta(2)+theta(3))*cos(theta(2)+theta(3)) + 2*m4*(l3 - lc4)^2*sin(theta(2)+theta(3))*cos(theta(2)+theta(3))...
     - 2*m4*l2^2*sin(theta(2))*cos(theta(2)) + 2*m4*(l3 - lc4)*l2*sin(theta(2))*sin(theta(2)+theta(3)) - 2*m4*(l3 - lc4)*l2*cos(theta(2))*cos(theta(2)+theta(3))...
     + 2*I4L*sin(theta(2)+theta(3))*cos(theta(2)+theta(3)) - 2*I4A*sin(theta(2)+theta(3))*cos(theta(2)+theta(3)) + 2*mL*l3^2*sin(theta(2)+theta(3))*cos(theta(2)+theta(3))...
     - 2*mL*l2^2*sin(theta(2))*cos(theta(2)) + 2*mL*l2*l3*sin(theta(2))*sin(theta(2)+theta(3)) - 2*mL*l2*l3*cos(theta(2))*cos(theta(2)+theta(3));
B12 =  2*m3*lc3^2*sin(theta(2)+theta(3))*cos(theta(2)+theta(3)) - 2*m3*l2*lc3*cos(theta(2))*cos(theta(2)+theta(3)) + 2*I3L*sin(theta(2)+theta(3))*cos(theta(2)+theta(3))...
     - 2*I3A*sin(theta(2)+theta(3))*cos(theta(2)+theta(3)) + 2*m4*(l3-lc4)^2*sin(theta(2)+theta(3))*cos(theta(2)+theta(3)) - 2*m4*(l3-lc4)*l2*cos(theta(2))*cos(theta(2)+theta(3))...
     + 2*I4L*sin(theta(2)+theta(3))*cos(theta(2)+theta(3)) - 2*I4A*sin(theta(2)+theta(3))*cos(theta(2)+theta(3)) + 2*mL*l3^2*sin(theta(2)+theta(3))*cos(theta(2)+theta(3))...
     - 2*mL*l2*l3*cos(theta(2))*cos(theta(2)+theta(3));
B15 =  I4A*sin(theta(2)+theta(3));
B16 =  I4A*sin(theta(2)+theta(3));
B23 = -I4A*sin(theta(2)+theta(3));
B24 = -2*m3*l2*lc3*cos(theta(3)) - 2*mL*l2*l3*cos(theta(3));
B33 = -I4A*sin(theta(2)+theta(3));
B41 =  I4A*sin(theta(2)+theta(3));
B42 =  I4A*sin(theta(2)+theta(3));
B = [B11, B12, 0, 0, B15, B16; 0, 0, B23, B24, 0, 0; 0, 0, B33, 0, 0, 0; B41, B42, 0, 0, 0, 0];

% Centrifugal Matrix
C21 = -(-m2*(l2-lc2)^2*sin(theta(2))*cos(theta(2)) + I2A*sin(theta(2))*cos(theta(2)) - I2L*sin(theta(2))*cos(theta(2)) - m3*l2^2*sin(theta(2))*cos(theta(2))...
     + m3*lc3^2*sin(theta(2)+theta(3))*cos(theta(2)+theta(3)) + m3*l2*lc3*sin(theta(2))*sin(theta(2)+theta(3)) - m3*l2*lc3*cos(theta(2))*cos(theta(2)+theta(3))  ...
     + I3L*sin(theta(2)+theta(3))*cos(theta(2)+theta(3)) - I3A*sin(theta(2)+theta(3))*cos(theta(2)+theta(3)) + m4*(l3-lc4)^2*sin(theta(2)+theta(3))*cos(theta(2)+theta(3))...
     - m4*l2^2*sin(theta(2))*cos(theta(2)) + m4*(l3-lc4)*l2*sin(theta(2))*sin(theta(2)+theta(3)) - m4*(l3-lc4)*l2*cos(theta(2))*cos(theta(2)+theta(3)) ...
     + I4L*sin(theta(2)+theta(3))*cos(theta(2)+theta(3)) - I4A*sin(theta(2)+theta(3))*cos(theta(2)+theta(3)) + mL*l3^2*sin(theta(2)+theta(3))*cos(theta(2)+theta(3))...
     - mL*l2^2*sin(theta(2))*cos(theta(2)) + mL*l2*l3*sin(theta(2))*sin(theta(2)+theta(3)) - mL*l2*l3*cos(theta(2))*cos(theta(2)+theta(3)));
C23 = -mL*lc3*l2*cos(theta(3)) - m4*l2*cos(theta(3))*(l3 - lc4) + mL*l2*l3*cos(theta(3));
C31 = -(m3*lc3^2*sin(theta(2)+theta(3))*cos(theta(2)+theta(3)) - m3*l2*lc3*cos(theta(2))*cos(theta(2)+theta(3)) + I3L*sin(theta(2)+theta(3))*cos(theta(2)+theta(3))...
      - I3A*sin(theta(2)+theta(3))*cos(theta(2)+theta(3)) + m4*(l3-lc4)^2*sin(theta(2)+theta(3))*cos(theta(2)+theta(3)) ...
      - m4*(l3-lc4)*l2*cos(theta(2))*cos(theta(2)+theta(3)) + I4L*sin(theta(2)+theta(3))*cos(theta(2)+theta(3)) - I4A*sin(theta(2)+theta(3))*cos(theta(2)+theta(3))... 
      + mL*l3^2*sin(theta(2)+theta(3))*cos(theta(2)+theta(3)) - mL*l2*l3*cos(theta(2))*cos(theta(2)+theta(3)));
C32 = m3*l2*lc3*cos(theta(3)) + mL*l2*l3*cos(theta(3));
C = [0, 0, 0, 0; C21, 0, C23, 0; C31, C32, 0, 0; 0, 0, 0, 0];

% Gravity Matrix

G2 = -g*(m2*(l2 - lc2)*cos(theta(2)) + m3*(l2*cos(theta(2)) - lc3*sin(theta(2)+theta(3))) + m4*(l2*cos(theta(2)) - (l3 - lc4)*sin(theta(2)+theta(3))) + mL*(l2*cos(theta(2)) - l3*sin(theta(2)+theta(3))) );
G3 = g*(m3*lc3*sin(theta(2)+theta(3)) + m4*(l3 - lc4)*sin(theta(2)+theta(3)) + mL*l3*sin(theta(2)+theta(3)) );

G = [0; G2; G3; 0];

%% Friction
% Friction = [0; 0; 0; 0];

Bv = [0.2119; 0.0457; 0.001; 0.008]; % Viscous coeffcients
Bc = [0.0838; 0.6701; 0.6156; 0.0275]; % Coulomb coeffcients

Friction = [Bv(1)*theta_d(1) + Bc(1)*sign(theta_d(1));...
             Bv(2)*theta_d(2) + Bc(2)*sign(theta_d(2));...
             Bv(3)*theta_d(3) + Bc(3)*sign(theta_d(3));...
             Bv(4)*theta_d(4) + Bc(4)*sign(theta_d(4))];  

%% Torque Computation (without Gravity)

B_signals = [theta_d(1) .* theta_d(2);...
             theta_d(1) .* theta_d(3);...
             theta_d(1) .* theta_d(4);...
             theta_d(2) .* theta_d(3);...
             theta_d(2) .* theta_d(4);...
             theta_d(3) .* theta_d(4);...
             ];

tau = M * theta_dd + B * B_signals + C * theta_d.^2 + G + Friction;
end

%%
